simulink model "Yellow_Fever_Model"  (R2022b)
settings: Solver=ode4  StartTime=0.0  StopTime=275  FixedStep=1  RelTol=1e-3
values from neighbouring files (symbols this model uses):
  A_w_0 = 0    [Cibernetica_project.m]
  E_v_0 = 0    [Cibernetica_project.m]
  E_w_0 = 0    [Cibernetica_project.m]
  I_v_0 = 1    [Cibernetica_project.m]
  N_v_0 = S_v_0 + I_v_0    (= 225001)    [Cibernetica_project.m]
  N_w_0 = S_w_0 + A_w_0 + I_w_0    (= 8001)    [Cibernetica_project.m]
  Par = [beta_1_fg beta_2_fg gamma_h_fg theta_fg b_h_fg b_v_fg a_fg delta_fg        alpha_fg epsilon_fg rho_fg sigma_fg mu_h_fg mu_v_fg sigma_v p_fg]    [Cibernetica_project_fg.m]
  S_v_0 = 0.225*10^6    (= 225000)    [Cibernetica_project.m]
  S_w_0 = 8000    [Cibernetica_project.m]
settings Model: Creator=angel  LastModifiedBy=angel
settings SolverCC: EnableFixedStepZeroCrossing=on

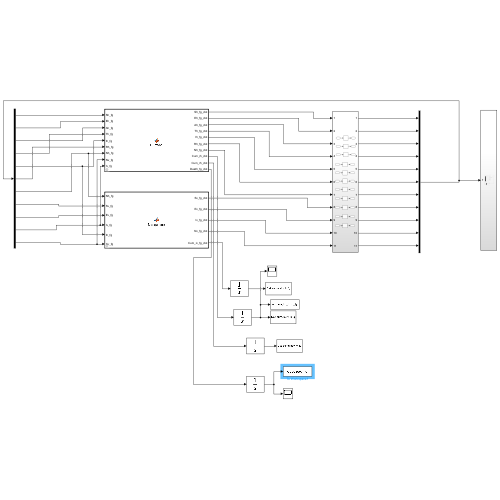
[thumbnail: Simulink's stored preview of the top-level diagram]
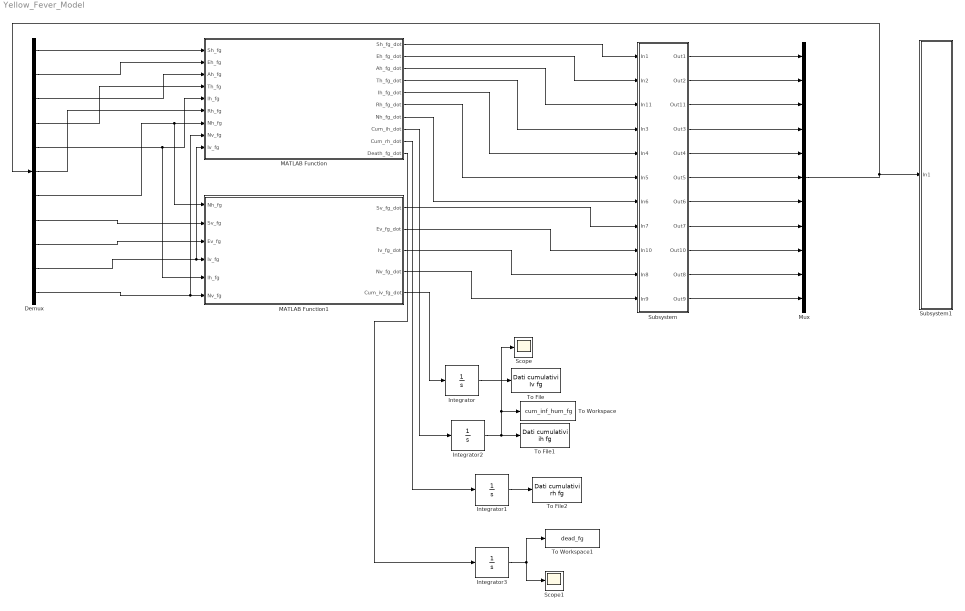
== system Yellow_Fever_Model ==
  Demux : Demux  Outputs=11
  Integrator{,1..3} (4 alike) : Integrator
  MATLAB Function : MATLAB Function  TreatAsAtomicUnit=on  mask{Par=Par}
      mask prompts: Par "Parametri del Sistema"
  MATLAB Function1 : MATLAB Function  TreatAsAtomicUnit=on  mask{Par=Par}
      mask prompts: Par "Parametri del Sistema"
  Mux : Mux  Inputs=11
  Scope : Scope
  Scope1 : Scope
  Subsystem : Subsystem
  Subsystem1 : Subsystem
  To File : ToFile  Filename=Dati cumulativi Iv fg  MatrixName=Cum_iv  SampleTime=1
  To File1 : ToFile  Filename=Dati cumulativi ih fg  MatrixName=Cum_ih  SampleTime=1
  To File2 : ToFile  Filename=Dati cumulativi rh fg  MatrixName=Cum_rh  SampleTime=1
  To Workspace : ToWorkspace  VariableName=cum_inf_hum_fg  SaveFormat=Timeseries  SampleTime=1
  To Workspace1 : ToWorkspace  VariableName=dead_fg  SampleTime=1
  wires:
  MATLAB Function/1(Sh_fg_dot) -> Subsystem/1(In1)
  MATLAB Function/2(Eh_fg_dot) -> Subsystem/2(In2)
  MATLAB Function/4(Th_fg_dot) -> Subsystem/4(In3)
  MATLAB Function/5(Ih_fg_dot) -> Subsystem/5(In4)
  MATLAB Function/6(Rh_fg_dot) -> Subsystem/6(In5)
  MATLAB Function/7(Nh_fg_dot) -> Subsystem/7(In6)
  MATLAB Function1/1(Sv_fg_dot) -> Subsystem/8(In7)
  MATLAB Function1/3(Iv_fg_dot) -> Subsystem/10(In8)
  MATLAB Function1/4(Nv_fg_dot) -> Subsystem/11(In9)
  Subsystem/1(Out1) -> Mux/1
  Subsystem/2(Out2) -> Mux/2
  Mux/1 -> Demux/1, Subsystem1/1(In1)
  Demux/1 -> MATLAB Function/1(Sh_fg)
  Demux/2 -> MATLAB Function/2(Eh_fg)
  MATLAB Function1/5(Cum_iv_fg_dot) -> Integrator/1
  MATLAB Function/8(Cum_ih_dot) -> Integrator2/1
  MATLAB Function/9(Cum_rh_dot) -> Integrator1/1
  Integrator/1 -> To File/1
  Integrator2/1 -> To Workspace/1, Scope/1, To File1/1
  Integrator1/1 -> To File2/1
  MATLAB Function1/2(Ev_fg_dot) -> Subsystem/9(In10)
  MATLAB Function/3(Ah_fg_dot) -> Subsystem/3(In11)
  Subsystem/3(Out11) -> Mux/3
  Subsystem/4(Out3) -> Mux/4
  Subsystem/5(Out4) -> Mux/5
  Subsystem/6(Out5) -> Mux/6
  Subsystem/7(Out6) -> Mux/7
  Subsystem/8(Out7) -> Mux/8
  Subsystem/9(Out10) -> Mux/9
  Subsystem/10(Out8) -> Mux/10
  Subsystem/11(Out9) -> Mux/11
  Demux/3 -> MATLAB Function/3(Ah_fg)
  Demux/4 -> MATLAB Function/4(Th_fg)
  Demux/5 -> MATLAB Function1/5(Ih_fg), MATLAB Function/5(Ih_fg)
  Demux/6 -> MATLAB Function/6(Rh_fg)
  Demux/7 -> MATLAB Function1/1(Nh_fg), MATLAB Function/7(Nh_fg)
  Demux/8 -> MATLAB Function1/2(Sv_fg)
  Demux/9 -> MATLAB Function1/3(Ev_fg)
  Demux/11 -> MATLAB Function/8(Nv_fg), MATLAB Function1/6(Nv_fg)
  Demux/10 -> MATLAB Function/9(Iv_fg), MATLAB Function1/4(Iv_fg)
  MATLAB Function/10(Death_fg_dot) -> Integrator3/1
  Integrator3/1 -> To Workspace1/1, Scope1/1

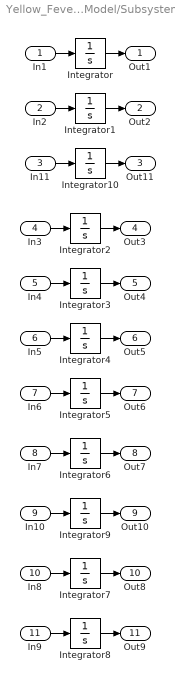
== system Yellow_Fever_Model/Subsystem ==
  In1 : Inport
  In2 : Inport  Port=2
  In11 : Inport  Port=3
  In3 : Inport  Port=4
  In4 : Inport  Port=5
  In5 : Inport  Port=6
  In6 : Inport  Port=7
  In7 : Inport  Port=8
  In10 : Inport  Port=9
  In8 : Inport  Port=10
  In9 : Inport  Port=11
  Integrator : Integrator  InitialCondition=S_w_0
  Integrator1 : Integrator  InitialCondition=E_w_0
  Integrator10 : Integrator  InitialCondition=A_w_0
  Integrator2 : Integrator
  Integrator3 : Integrator
  Integrator4 : Integrator
  Integrator5 : Integrator  InitialCondition=N_w_0
  Integrator6 : Integrator  InitialCondition=S_v_0
  Integrator7 : Integrator  InitialCondition=I_v_0
  Integrator8 : Integrator  InitialCondition=N_v_0
  Integrator9 : Integrator  InitialCondition=E_v_0
  Out1 : Outport
  Out2 : Outport  Port=2
  Out11 : Outport  Port=3
  Out3 : Outport  Port=4
  Out4 : Outport  Port=5
  Out5 : Outport  Port=6
  Out6 : Outport  Port=7
  Out7 : Outport  Port=8
  Out10 : Outport  Port=9
  Out8 : Outport  Port=10
  Out9 : Outport  Port=11
  wires:
  Integrator1/1 -> Out2/1
  In8/1 -> Integrator7/1
  In2/1 -> Integrator1/1
  In1/1 -> Integrator/1
  Integrator/1 -> Out1/1
  Integrator7/1 -> Out8/1
  In3/1 -> Integrator2/1
  Integrator3/1 -> Out4/1
  Integrator8/1 -> Out9/1
  In4/1 -> Integrator3/1
  Integrator2/1 -> Out3/1
  In9/1 -> Integrator8/1
  Integrator5/1 -> Out6/1
  In7/1 -> Integrator6/1
  In6/1 -> Integrator5/1
  Integrator4/1 -> Out5/1
  In5/1 -> Integrator4/1
  Integrator6/1 -> Out7/1
  Integrator9/1 -> Out10/1
  In10/1 -> Integrator9/1
  In11/1 -> Integrator10/1
  Integrator10/1 -> Out11/1

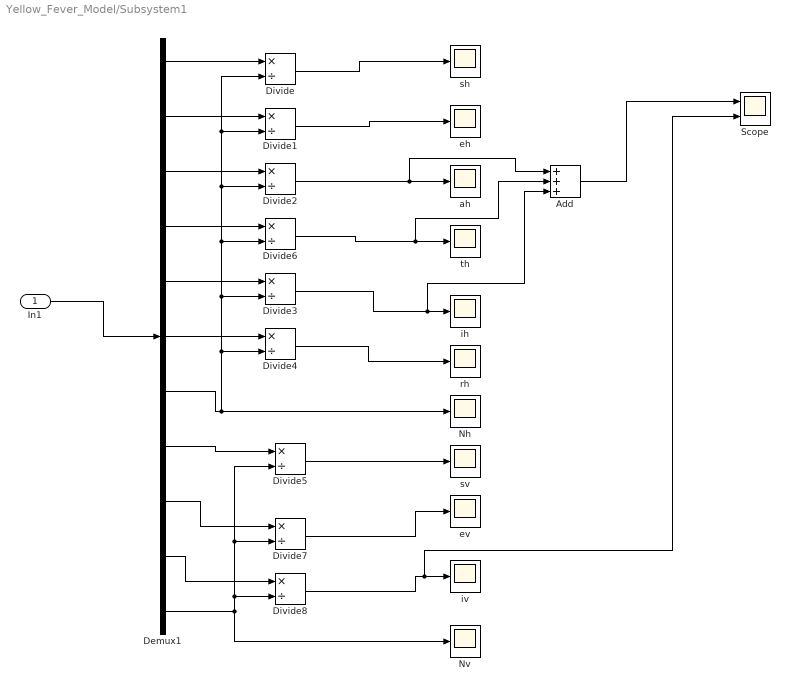
== system Yellow_Fever_Model/Subsystem1 ==
  In1 : Inport
  Add : Sum  Inputs=+++
  Demux1 : Demux  Outputs=11
  Divide{,1..8} (9 alike) : Product  Inputs=*/
  Nh : Scope
  Nv : Scope
  Scope : Scope  NumInputPorts=2
  ah : Scope
  eh : Scope
  ev : Scope
  ih : Scope
  iv : Scope
  rh : Scope
  sh : Scope
  sv : Scope
  th : Scope
  wires:
  In1/1 -> Demux1/1
  Divide/1 -> sh/1
  Divide1/1 -> eh/1
  Divide2/1 -> Add/1, ah/1
  Divide5/1 -> sv/1
  Divide7/1 -> ev/1
  Demux1/10 -> Divide8/1
  Demux1/9 -> Divide7/1
  Demux1/8 -> Divide5/1
  Divide8/1 -> Scope/2, iv/1
  Demux1/11 -> Nv/1, Divide8/2, Divide7/2, Divide5/2
  Demux1/6 -> Divide4/1
  Demux1/5 -> Divide3/1
  Demux1/1 -> Divide/1
  Demux1/2 -> Divide1/1
  Demux1/3 -> Divide2/1
  Demux1/4 -> Divide6/1
  Demux1/7 -> Divide4/2, Divide3/2, Divide6/2, Divide2/2, Divide1/2, Divide/2, Nh/1
  Divide6/1 -> Add/2, th/1
  Divide3/1 -> ih/1, Add/3
  Divide4/1 -> rh/1
  Add/1 -> Scope/1

== matlab function Yellow_Fever_Model/MATLAB Function1 ==
  data: Nh_fg input; Sv_fg input; Ev_fg input; Iv_fg input; Ih_fg input; Sv_fg_dot output; Ev_fg_dot output; Iv_fg_dot output; Nv_fg input; Nv_fg_dot output; Par parameter; Cum_iv_fg_dot output
function [Sv_fg_dot, Ev_fg_dot, Iv_fg_dot, Nv_fg_dot, Cum_iv_fg_dot]= Mosquitoes(Nh_fg,Sv_fg, ...
    Ev_fg, Iv_fg, Ih_fg, Nv_fg, Par)
%% Parametri

beta_1_fg = Par(1);
beta_2_fg = Par(2);
gamma_h_fg = Par(3); 
theta_fg  = Par(4);
b_h_fg = Par(5);
b_v_fg = Par(6);
a_fg = Par(7);
delta_fg = Par(8);
alpha_fg = Par(9);
epsilon_fg = Par(10);
rho_fg = Par(11); 
sigma_fg = Par(12); 
mu_h_fg = Par(13);
mu_v_fg = Par(14);
sigma_v = Par(15);
p_fg = Par(16);

lambda_hv = (a_fg*beta_2_fg*Sv_fg*Ih_fg)/Nh_fg; % infettività dagli umani
%% Dinamica

Sv_fg_dot = b_v_fg*Nv_fg - lambda_hv - mu_v_fg*Sv_fg;
Ev_fg_dot = lambda_hv - (mu_v_fg + sigma_v)*Ev_fg;
Iv_fg_dot = sigma_v*Ev_fg - mu_v_fg*Iv_fg;
Nv_fg_dot = (b_v_fg - mu_v_fg)*Nv_fg;
Cum_iv_fg_dot = sigma_v*Ev_fg;

% Sv_fg_dot = b_v_fg - a_fg*beta_2_fg*Sv_fg*Ih_fg - mu_v_fg*Sv_fg;
% Iv_fg_dot = a_fg*beta_2_fg*Sv_fg*Ih_fg - mu_v_fg*Iv_fg;
% Nv_fg_dot = (b_v_fg - mu_v_fg)*Nv_fg;

== matlab function Yellow_Fever_Model/MATLAB Function ==
  data: Sh_fg input; Sh_fg_dot output; Eh_fg input; Ah_fg input; Th_fg input; Ih_fg input; Rh_fg input; Nh_fg input; Nv_fg input; Iv_fg input; Eh_fg_dot output; Ah_fg_dot output; Th_fg_dot output; Ih_fg_dot output; Rh_fg_dot output; Nh_fg_dot output; Par parameter; Cum_ih_dot output; Cum_rh_dot output; Death_fg_dot output
function [Sh_fg_dot,Eh_fg_dot,Ah_fg_dot,Th_fg_dot,Ih_fg_dot,Rh_fg_dot,Nh_fg_dot,Cum_ih_dot,Cum_rh_dot,Death_fg_dot] = ...
Humans(Sh_fg,Eh_fg,Ah_fg,Th_fg,Ih_fg,Rh_fg,Nh_fg, Nv_fg,Iv_fg, Par)
%% Parametri

beta_1_fg = Par(1);
beta_2_fg = Par(2);
gamma_h_fg = Par(3); 
theta_fg  = Par(4);
b_h_fg = Par(5);
b_v_fg = Par(6);
a_fg = Par(7);
delta_fg = Par(8);
alpha_fg = Par(9);
epsilon_fg = Par(10);
rho_fg = Par(11); 
sigma_fg = Par(12); 
mu_h_fg = Par(13);
mu_v_fg = Par(14);
sigma_v = Par(15);
p_fg = Par(16);

%LAMBDA = sigma_fg*Nh_fg;
LAMBDA = 0;
lambda_vh = (a_fg*beta_1_fg*Sh_fg*Iv_fg)/Nv_fg; % infettività dalle 
                                                    % zanzare

%% Dinamica Umani

Sh_fg_dot = b_h_fg*Nh_fg + (1-rho_fg)*LAMBDA - lambda_vh - epsilon_fg*Sh_fg...
    - mu_h_fg*Sh_fg;
Eh_fg_dot = lambda_vh - gamma_h_fg*Eh_fg - mu_h_fg*Eh_fg;
Ah_fg_dot = p_fg*gamma_h_fg*Eh_fg - delta_fg*Ah_fg - mu_h_fg*Ah_fg;
Th_fg_dot = (1-p_fg)*theta_fg*gamma_h_fg*Eh_fg - delta_fg*Th_fg - (mu_h_fg + alpha_fg)...
    *Th_fg;
Ih_fg_dot = (1-p_fg)*(1-theta_fg)*gamma_h_fg*Eh_fg - delta_fg*Ih_fg - (mu_h_fg + alpha_fg)...
    *Ih_fg;
Rh_fg_dot = delta_fg*Th_fg + delta_fg*Ih_fg + rho_fg*LAMBDA + epsilon_fg*Sh_fg...
    - mu_h_fg*Rh_fg;
Nh_fg_dot = LAMBDA + (b_h_fg - mu_h_fg)*Nh_fg - alpha_fg*Ih_fg - alpha_fg*Th_fg;

Cum_ih_dot = gamma_h_fg*(Eh_fg);
Cum_rh_dot = delta_fg*Th_fg + delta_fg*Ih_fg + delta_fg*Ah_fg + rho_fg*LAMBDA + epsilon_fg*Sh_fg;
Death_fg_dot = alpha_fg*(Ih_fg + Th_fg) + mu_h_fg*(Sh_fg + Eh_fg_dot + ...
    Ah_fg + Th_fg + Ih_fg + Rh_fg);

% Sh_fg_dot = b_h_fg + (1-rho_fg)*sigma_fg - a_fg*beta_1_fg*Sh_fg*Iv_fg - epsilon_fg*Sh_fg...
%     - mu_h_fg*Sh_fg;
% Eh_fg_dot = a_fg*beta_1_fg*Sh_fg*Iv_fg - gamma_h_fg*Eh_fg - mu_h_fg*Eh_fg;
% Th_fg_dot = theta_fg*gamma_h_fg*Eh_fg - delta_fg*Th_fg - (mu_h_fg + alpha_fg)...
%     *Th_fg;
% Ih_fg_dot = (1-theta_fg)*gamma_h_fg*Eh_fg - delta_fg*Ih_fg - (mu_h_fg + alpha_fg)...
%     *Ih_fg;
% Rh_fg_dot = delta_fg*Th_fg + delta_fg*Ih_fg + rho_fg*sigma_fg + epsilon_fg*Sh_fg...
%     - mu_h_fg*Rh_fg;
% Nh_fg_dot = LAMBDA + (b_h_fg - mu_h_fg)*Nh_fg - alpha_fg*Ih_fg - alpha_fg*Th_fg;
